simulink model "tdhdkPI"  (R2016a)
settings: Solver=VariableStepAuto  StartTime=0.0  StopTime=10  RelTol=1e-3
undefined symbols (not defined in the file): bequiv, Jequiv, Kb, Ki1, Kp1, Kt, Ktach, La, n, r, Ra, Z
libraries: simulink x1
settings Model: Creator=Tuan  LastModifiedBy=Tuan

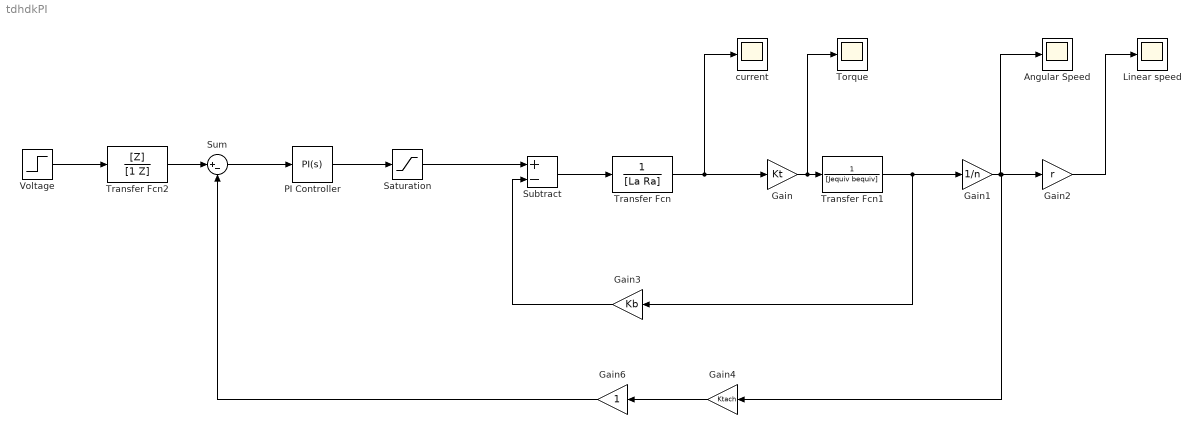
== system tdhdkPI ==
  Angular Speed : Scope
  Gain : Gain  Gain=Kt
  Gain1 : Gain  Gain=1/n
  Gain2 : Gain  Gain=r
  Gain3 : Gain  Gain=Kb
  Gain4 : Gain  Gain=Ktach
  Gain6 : Gain
  Linear speed : Scope
  PI Controller : simulink/Continuous/PID Controller  Controller=PI  TimeDomain=Continuous-time  SampleTime=-1  IntegratorMethod=Forward Euler  FilterMethod=Forward Euler  Form=Parallel  UseFilter=on  ControllerParametersSource=internal  P=Kp1  I=Ki1  D=0  N=100  InitialConditionSource=internal  InitialConditionForIntegrator=0  InitialConditionForFilter=0  ExternalReset=none  LimitOutput=off  UpperSaturationLimit=inf  LowerSaturationLimit=-inf  LinearizeAsGain=on  AntiWindupMode=none  Kb=1  TrackingMode=off  Kt=1  PParamMin=[]  PParamMax=[]  IParamMin=[]  IParamMax=[]  DParamMin=[]  DParamMax=[]  NParamMin=[]  NParamMax=[]  KbParamMin=[]  KbParamMax=[]  KtParamMin=[]  KtParamMax=[]  POutMin=[]  POutMax=[]  IOutMin=[]  IOutMax=[]  DOutMin=[]  DOutMax=[]  NOutMin=[]  NOutMax=[]  KbOutMin=[]  KbOutMax=[]  KtOutMin=[]  KtOutMax=[]  IntegratorOutMin=[]  IntegratorOutMax=[]  FilterOutMin=[]  FilterOutMax=[]  SumOutMin=[]  SumOutMax=[]  SumI1OutMin=[]  SumI1OutMax=[]  SumI2OutMin=[]  SumI2OutMax=[]  SumI3OutMin=[]  SumI3OutMax=[]  SumDOutMin=[]  SumDOutMax=[]  SaturationOutMin=[]  SaturationOutMax=[]  IntegratorContinuousStateAttributes=''  IntegratorStateMustResolveToSignalObject=off  IntegratorRTWStateStorageClass=Auto  FilterContinuousStateAttributes=''  FilterStateMustResolveToSignalObject=off  FilterRTWStateStorageClass=Auto  DifferentiatorICPrevScaledInput=0  DifferentiatorOutMin=[]  DifferentiatorOutMax=[]
  Saturation : Saturate  UpperLimit=20  LowerLimit=-20
  Subtract : Sum  Inputs=+-
  Sum : Sum  Inputs=|+-
  Torque : Scope
  Transfer Fcn : TransferFcn  Denominator=[La Ra]
  Transfer Fcn1 : TransferFcn  Denominator=[Jequiv bequiv]
  Transfer Fcn2 : TransferFcn  Numerator=[Z]  Denominator=[1 Z]
  Voltage : Step  Time=0  After=12  SampleTime=0
  current : Scope
  wires:
  Saturation/1 -> Subtract/1
  Subtract/1 -> Transfer Fcn/1
  Transfer Fcn/1 -> current/1, Gain/1
  Transfer Fcn1/1 -> Gain3/1, Gain1/1
  Gain1/1 -> Gain4/1, Gain2/1, Angular Speed/1
  Gain2/1 -> Linear speed/1
  Gain3/1 -> Subtract/2
  Gain/1 -> Torque/1, Transfer Fcn1/1
  Gain4/1 -> Gain6/1
  Sum/1 -> PI Controller/1
  PI Controller/1 -> Saturation/1
  Gain6/1 -> Sum/2
  Voltage/1 -> Transfer Fcn2/1
  Transfer Fcn2/1 -> Sum/1
